simulink model "ball_detection"  (R2020a)
settings: Solver=FixedStepAuto  StartTime=0.0  StopTime=10.0  RelTol=1e-3
model workspace (MAT data in the model file):
  SL_ROS_VariableLengthArrays_MaxSizes.CommonInfo.ArrayTruncateAction = 'EmitWarning'
  SL_ROS_VariableLengthArrays_MaxSizes.MsgTypeMap = containers.Map
  SL_ROS_VariableLengthArrays_MaxSizes.MsgTypeMap.serialization.keys = {'sensor_msgs/Image'}
  SL_ROS_VariableLengthArrays_MaxSizes.MsgTypeMap.serialization.values{1}(1).PropertyName = 'Data'
  SL_ROS_VariableLengthArrays_MaxSizes.MsgTypeMap.serialization.values{1}(1).DataType = 'uint8'
  SL_ROS_VariableLengthArrays_MaxSizes.MsgTypeMap.serialization.values{1}(1).MaxLength = 3121200
  SL_ROS_VariableLengthArrays_MaxSizes.MsgTypeMap.serialization.values{1}(2).PropertyName = 'Encoding'
  SL_ROS_VariableLengthArrays_MaxSizes.MsgTypeMap.serialization.values{1}(2).DataType = 'uint8'
  SL_ROS_VariableLengthArrays_MaxSizes.MsgTypeMap.serialization.values{1}(2).MaxLength = 128
  SL_ROS_VariableLengthArrays_MaxSizes.MsgTypeMap.serialization.uniformity = 0
  SL_ROS_VariableLengthArrays_MaxSizes.MsgTypeMap.serialization.keyType = 'char'
  SL_ROS_VariableLengthArrays_MaxSizes.MsgTypeMap.serialization.valueType = 'any'
undefined symbols (not defined in the file): gray
libraries: robotlib x2
settings Model: Creator=shiva  LastModifiedBy=shiva
settings OptimizationCC: ZeroExternalMemoryAtStartup=off  ZeroInternalMemoryAtStartup=off
settings RTWCC: TargetLang=C++
settings GRTTargetCC: TargetLangStandard=C++03 (ISO)  MultiInstanceERTCode=on  CodeInterfacePackaging=C++ class

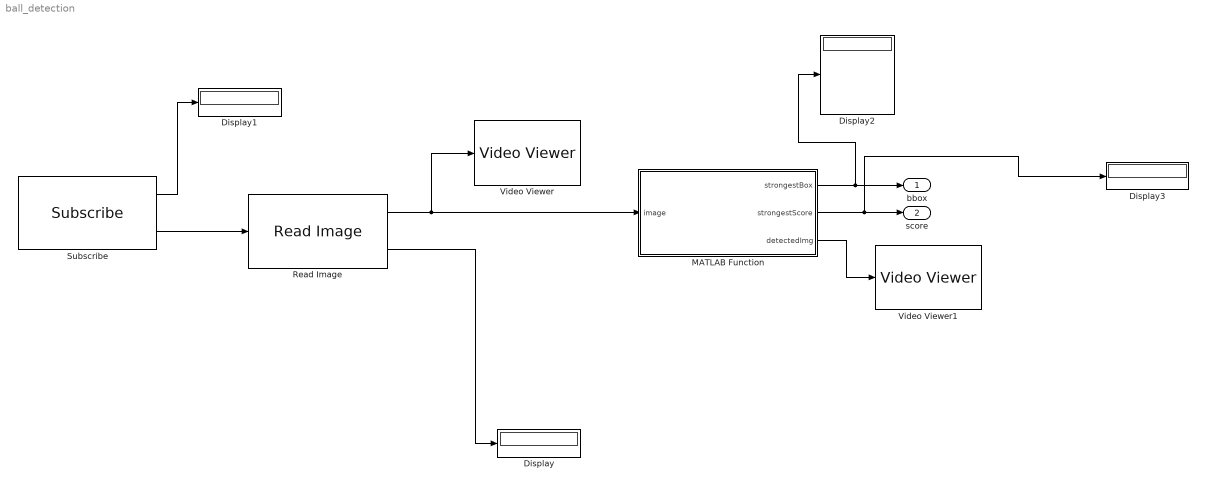
== system ball_detection ==
  Display{,1..3} (4 alike) : Display
  MATLAB Function : MATLAB Function  TreatAsAtomicUnit=on
  Read Image : robotlib/Read Image  MaximumImageSize=[1020, 1020]  ImageEncoding=rgb8  ShowAlphaOutput=off  ShowErrorCodeOutput=on  VariableSizeOutputs=off
      settings: SourceProductBaseCode=RR
  Subscribe : robotlib/Subscribe  topicSource=Select from ROS network  topic=/robot_sensor/camera/image_raw  messageType=sensor_msgs/Image  sampleTime=-1  messageQueueLength=1
  Video Viewer : VideoViewer  colormapValue=gray(256)  FigPos=[121 653 428 297]
  Video Viewer1 : VideoViewer  colormapValue=gray(256)  FigPos=[1199 792 418 304]
  bbox : Outport
  score : Outport  Port=2
  wires:
  Subscribe/2 -> Read Image/1
  Read Image/2 -> Display/1
  Read Image/1 -> MATLAB Function/1(image), Video Viewer/1
  Subscribe/1 -> Display1/1
  MATLAB Function/2(strongestScore) -> Display3/1, score/1
  MATLAB Function/1(strongestBox) -> Display2/1, bbox/1
  MATLAB Function/3(detectedImg) -> Video Viewer1/1

== matlab function ball_detection/MATLAB Function ==
  data: image input; strongestBox output; strongestScore output; detectedImg output
function [strongestBox, strongestScore, detectedImg] = yolov2_detect(image)
strongestBox = zeros(1, 4);
strongestScore = 0;

imageResized = imresize(image,[224, 224]);
detectedImg = imageResized;
persistent yolov2Obj;

if isempty(yolov2Obj)
    yolov2Obj = coder.loadDeepLearningNetwork('yoloResNet50_det.mat');
end

[bboxes, scores] = yolov2Obj.detect(imageResized,'Threshold',0.1);

if(~isempty(strongestBox))
    [strongestBox, strongestScore] = selectStrongestBbox(bboxes,scores,...
        'RatioType','Union',...
        'OverlapThreshold',0.5);
    strongestBox = strongestBox(1, :);
    strongestScore = double(strongestScore(1));
    
    detectedImg = insertObjectAnnotation(imageResized,'rectangle',...
        strongestBox,strongestScore, 'Color', [229, 0, 0]);
end
end
